simulink model "SOFCI_integral_simulation"  (R2022b)
settings: Solver=FixedStepAuto  StartTime=0.0  StopTime=10  RelTol=1e-3
values from neighbouring files (symbols this model uses):
  b = 0    [step_response_nominal.m]
  K_aug = [K_SF K_int]    [step_response_nominal.m]    (also in step_response_our.m)
  L = 0.23e-3    (= 0.00023)    [step_response_nominal.m]
  R = 3.85    [step_response_nominal.m]
  Stepsize = 0.5    [step_response_nominal.m]    (also in step_response_our.m)
  Tcomp = 0.0005*Ts*14    (= 7e-06)    [step_response_nominal.m]    (also in step_response_our.m)
  Ts = 0.001    [step_response_nominal.m]    (also in step_response_our.m)
  Tss = 1/20000    (= 5e-05)    [step_response_nominal.m]    (also in step_response_our.m = 0.0001)
undefined symbols (not defined in the file or in its folder): A_d, B_d, C_d, K_int, K_SF, L_Pred, N
settings Model: Creator=Alex Zhen  LastModifiedBy=lenovo
settings SolverCC: ZeroCrossControl=DisableAll  ZeroCrossAlgorithm=Adaptive
settings DebuggingCC: IgnoredZcDiagnostic=none

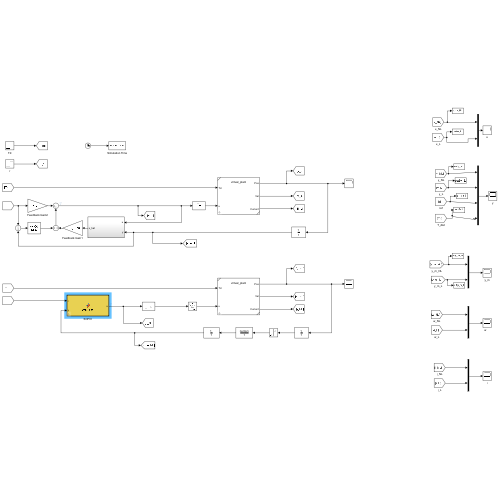
[thumbnail: Simulink's stored preview of the top-level diagram]
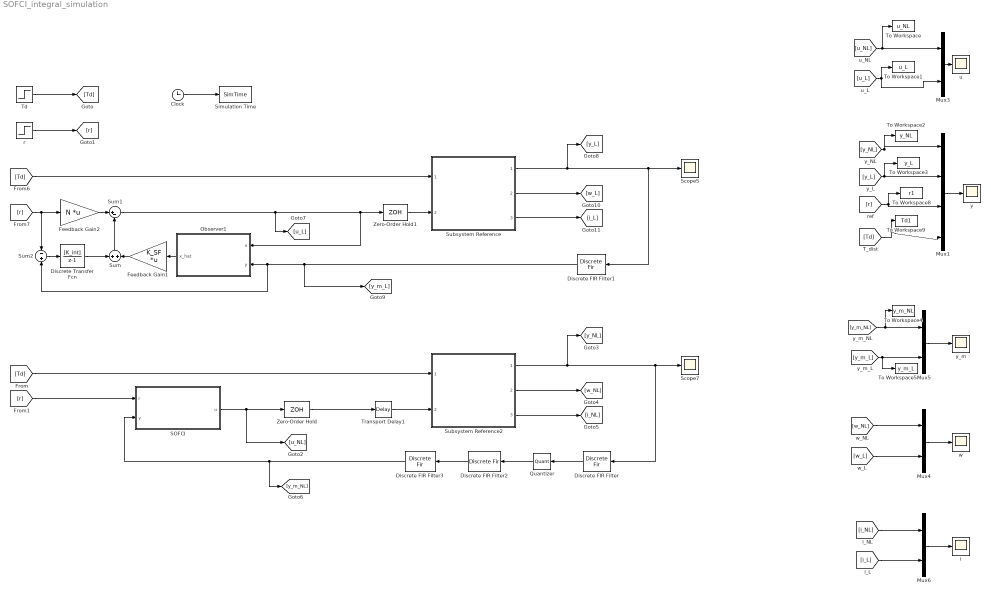
== system SOFCI_integral_simulation ==
  Clock : Clock
  Discrete Transfer Fcn : DiscreteTransferFcn  Numerator=[K_int]  Denominator=[1 -1]  SampleTime=Ts
  Discrete FIR Filter : DiscreteFir  Coefficients=[1]  SampleTime=Tss
  Discrete FIR Filter1 : DiscreteFir  Coefficients=[1]  SampleTime=Ts
  Discrete FIR Filter2 : DiscreteFir  Coefficients=[0.25 0.25 0.25 0.25]
  Discrete FIR Filter3 : DiscreteFir  Coefficients=[1]  SampleTime=Ts
  Feedback Gain1 : Gain  Gain=K_SF  Multiplication=Matrix(K*u)
  Feedback Gain2 : Gain  Gain=N  Multiplication=Matrix(K*u)
  Mux1 : Mux
  Mux{3..6} (4 alike) : Mux  Inputs=2
  Observer1 : Subsystem
  Quantizer : Quantizer  QuantizationInterval=encoder_resolution
  SOFCI : MATLAB Function  TreatAsAtomicUnit=on  mask{A=A_d, B=B_d, C=C_d, K=K_aug, L=L_Pred, N=N}
  Scope5 : Scope
  Scope7 : Scope
  Simulation Time : ToWorkspace  VariableName=SimTime  SampleTime=-1
  Subsystem Reference : Subsystem  ReferencedSubsystem=virtual_plant  L=L  K_m=K_m  J_pend=J_pend  b=b  V_s=V_s  R=R  K_pend=K_pend  K_sin=K_sin  K_g=K_g  linear_mode=Linear
  Subsystem Reference2 : Subsystem  ReferencedSubsystem=virtual_plant  L=L  K_m=K_m  J_pend=J_pend  b=b  V_s=V_s  R=R  K_pend=K_pend  K_sin=K_sin  K_g=K_g  linear_mode=Nonlinear
  Sum : Sum  Inputs=+|+
  Sum1 : Sum  Inputs=|+-
  Sum2 : Sum  Inputs=-|+
  Td : Step  Time=5  After=0.05  SampleTime=0
  To Workspace : ToWorkspace  VariableName=u_NL  SampleTime=Ts
  To Workspace1 : ToWorkspace  VariableName=u_L  SampleTime=Ts
  To Workspace2 : ToWorkspace  VariableName=y_NL  SampleTime=Ts
  To Workspace3 : ToWorkspace  VariableName=y_L  SampleTime=Ts
  To Workspace4 : ToWorkspace  VariableName=y_m_NL  SampleTime=Ts
  To Workspace5 : ToWorkspace  VariableName=y_m_L  SampleTime=Ts
  To Workspace8 : ToWorkspace  VariableName=r1  SampleTime=Ts
  To Workspace9 : ToWorkspace  VariableName=Td1  SampleTime=Ts
  Transport Delay1 : TransportDelay  DelayTime=Tcomp  BufferSize=4096  PadeOrder=2
  Zero-Order Hold : ZeroOrderHold  SampleTime=Ts
  Zero-Order Hold1 : ZeroOrderHold  SampleTime=Ts
  i : Scope
  r : Step  After=Stepsize  SampleTime=Ts
  u : Scope
  "w\t" : Scope
  y : Scope
  y_m : Scope
  wires:
  Discrete FIR Filter3/1 -> SOFCI/2(y), [y_m_NL]
  Feedback Gain2/1 -> Sum1/1
  Subsystem Reference2/1 -> [y_NL], Scope7/1, Discrete FIR Filter/1
  Observer1/1(x_hat) -> Feedback Gain1/1
  Subsystem Reference/2 -> [w_L]
  Transport Delay1/1 -> Subsystem Reference2/2
  [Td] -> Subsystem Reference/1
  Discrete FIR Filter/1 -> Quantizer/1
  Feedback Gain1/1 -> Sum/2
  Zero-Order Hold/1 -> Transport Delay1/1
  Subsystem Reference/1 -> Scope5/1, Discrete FIR Filter1/1, [y_L]
  Quantizer/1 -> Discrete FIR Filter2/1
  Subsystem Reference/3 -> [i_L]
  Subsystem Reference2/3 -> [i_NL]
  Discrete FIR Filter2/1 -> Discrete FIR Filter3/1
  [r] -> SOFCI/1(r)
  r/1 -> [r]
  Td/1 -> [Td]
  Sum1/1 -> [u_L], Observer1/1(u), Zero-Order Hold1/1
  Clock/1 -> Simulation Time/1
  Subsystem Reference2/2 -> [w_NL]
  Zero-Order Hold1/1 -> Subsystem Reference/2
  [Td] -> Subsystem Reference2/1
  SOFCI/1(u) -> Zero-Order Hold/1, [u_NL]
  [i_NL] -> Mux6/1
  Mux6/1 -> i/1
  [r] -> To Workspace8/1, Mux1/3
  [y_m_L] -> To Workspace5/1, Mux5/2
  [w_L] -> Mux4/2
  [i_L] -> Mux6/2
  Mux3/1 -> u/1
  Mux4/1 -> "w\t"/1
  [y_L] -> To Workspace3/1, Mux1/2
  [y_NL] -> To Workspace2/1, Mux1/1
  Mux1/1 -> y/1
  [u_L] -> To Workspace1/1, Mux3/2
  [u_NL] -> To Workspace/1, Mux3/1
  Mux5/1 -> y_m/1
  [y_m_NL] -> To Workspace4/1, Mux5/1
  [w_NL] -> Mux4/1
  [Td] -> To Workspace9/1, Mux1/4
  Sum2/1 -> Discrete Transfer Fcn/1
  Discrete Transfer Fcn/1 -> Sum/1
  Discrete FIR Filter1/1 -> [y_m_L], Sum2/2, Observer1/2(y)
  [r] -> Feedback Gain2/1, Sum2/1
  Sum/1 -> Sum1/2

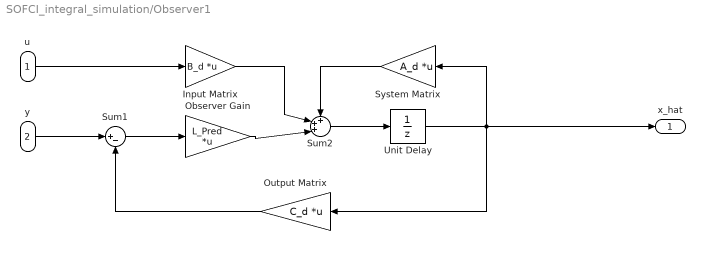
== system SOFCI_integral_simulation/Observer1 ==
  u : Inport
  y : Inport  Port=2
  Input Matrix : Gain  Gain=B_d  Multiplication=Matrix(K*u)
  Observer Gain : Gain  Gain=L_Pred  Multiplication=Matrix(K*u)
  Output Matrix : Gain  Gain=C_d  Multiplication=Matrix(K*u)
  Sum1 : Sum  Inputs=|+-
  Sum2 : Sum  Inputs=+++|
  System Matrix : Gain  Gain=A_d  Multiplication=Matrix(K*u)
  Unit Delay : UnitDelay  SampleTime=Ts  HasFrameUpgradeWarning=on
  x_hat : Outport
  wires:
  Sum1/1 -> Observer Gain/1
  System Matrix/1 -> Sum2/1
  Sum2/1 -> Unit Delay/1
  Output Matrix/1 -> Sum1/2
  Input Matrix/1 -> Sum2/2
  Observer Gain/1 -> Sum2/3
  u/1 -> Input Matrix/1
  Unit Delay/1 -> Output Matrix/1, x_hat/1, System Matrix/1
  y/1 -> Sum1/1

== matlab function SOFCI_integral_simulation/SOFCI ==
  data: r input; u output; y input; A parameter; B parameter; C parameter; K parameter; L parameter; N parameter
function u = controller(r,y,A, B, C, K, L, N)

persistent xhat xint;  %memory for the state

  if isempty(xhat)  %local variable initialization
      n=size(L,1);
        xhat=zeros(n,1); 
      m = size(K,2)-n;
        xint=zeros(m,1);  
  end
xaug=[xhat; xint]; %Augmented state include the state for the integrator
%u = -K*xaug+N*r; %Control computation with integral action 
u_unsat = -K*xaug+N*r; %Control computation with integral action 
u= sign(u_unsat)*min(1,abs(u_unsat));
%DAC(u) send out control here to minimize computation delay
%Update the next state next
xhat = (A-L*C)*xhat + B*u + L*y;
xint = xint+ y-r;
